simulink model "Progetto_3B_simulink"  (R2019b)
settings: Solver=VariableStepAuto  StartTime=0.0  StopTime=10.0  RelTol=1e-3
values from neighbouring files (symbols this model uses):
  A_n = 0.05    [Progetto_3B.m]
  C_d = (2.2*pi^2)    (= 21.7131296824)    [Progetto_3B.m]
  D = 0    [Progetto_3B.m]
  eta = 0.65    [Progetto_3B.m]
  omega_n = 1500    [Progetto_3B.m]
  R_0 = 35    [Progetto_3B.m]
  u_ = ((x_1/(x_2*abs(x_2))- R_0) / C_d); u_    [Progetto_3B.m]
  x_1 = 10    [Progetto_3B.m]
  x_2 = 5    [Progetto_3B.m]
  y_notlin = -eta*x_1*x_2    (= -32.5)    [Progetto_3B.m]
undefined symbols (not defined in the file or in its folder): N
libraries: cstblocks x2
settings Model: Creator=Hiari  LastModifiedBy=Hiari

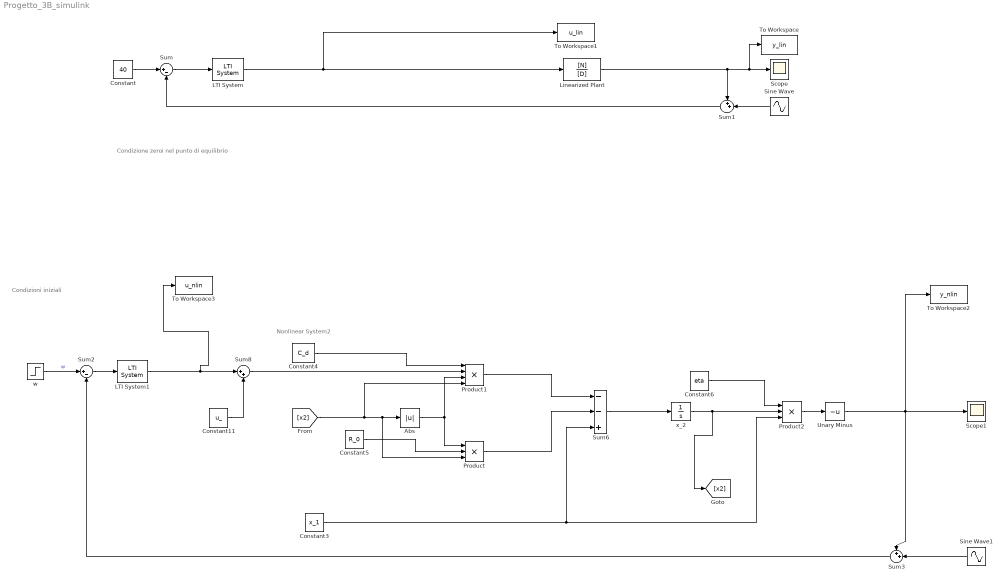
== system Progetto_3B_simulink ==
  note: Nonlinear
      | System2
  note: Condizione zeroi nel punto di equilibrio
  note: Condizioni iniziali
  Abs : Abs
  Constant : Constant  Value=40
  Constant11 : Constant  Value=u_
  Constant3 : Constant  Value=x_1
  Constant4 : Constant  Value=C_d  VectorParams1D=off
  Constant5 : Constant  Value=R_0
  Constant6 : Constant  Value=eta
  LTI System : cstblocks/LTI System  sys=R  IC=[]
  LTI System1 : cstblocks/LTI System  sys=R  IC=[]
  Linearized Plant : TransferFcn  Numerator=[N]  Denominator=[D]
  Product : Product  Inputs=3
  Product1 : Product  Inputs=4
  Product2 : Product  Inputs=3
  Scope : Scope
  Scope1 : Scope
  Sine Wave : Sin  Amplitude=A_n  Frequency=omega_n  SampleTime=0
  Sine Wave1 : Sin  Amplitude=A_n  Frequency=omega_n  SampleTime=0
  Sum : Sum  Inputs=|+-
  Sum1 : Sum  Inputs=++|
  Sum2 : Sum  Inputs=|+-
  Sum3 : Sum  Inputs=++|
  Sum6 : Sum  Inputs=--+
  Sum8 : Sum  Inputs=|++
  To Workspace : ToWorkspace  VariableName=y_lin  SaveFormat=Timeseries  SampleTime=-1
  To Workspace1 : ToWorkspace  VariableName=u_lin  SaveFormat=Timeseries  SampleTime=-1
  To Workspace2 : ToWorkspace  VariableName=y_nlin  SaveFormat=Timeseries  SampleTime=-1
  To Workspace3 : ToWorkspace  VariableName=u_nlin  SaveFormat=Timeseries  SampleTime=-1
  Unary Minus : UnaryMinus
  w : Step  Time=2  Before=y_notlin  After=y_notlin + 0.02  SampleTime=0
  "x_2 " : Integrator  InitialCondition=x_2
  wires:
  Linearized Plant/1 -> To Workspace/1, Scope/1, Sum1/1
  LTI System/1 -> To Workspace1/1, Linearized Plant/1
  Sum/1 -> LTI System/1
  Sine Wave/1 -> Sum1/2
  Sum1/1 -> Sum/2
  Constant/1 -> Sum/1
  Sum2/1 -> LTI System1/1
  Sum3/1 -> Sum2/2
  Constant3/1 -> Product2/3, Sum6/3
  Product2/1 -> Unary Minus/1
  Constant6/1 -> Product2/1
  Constant5/1 -> Product/2
  Abs/1 -> Product/1, Product1/3
  [x2] -> Abs/1, Product/3, Product1/4
  Sum6/1 -> "x_2 "/1
  Product/1 -> Sum6/2
  Product1/1 -> Sum6/1
  Constant4/1 -> Product1/1
  LTI System1/1 -> Sum8/1, To Workspace3/1
  "x_2 "/1 -> [x2], Product2/2
  Sum8/1 -> Product1/2
  Unary Minus/1 -> Sum3/1, To Workspace2/1, Scope1/1
  Constant11/1 -> Sum8/2
  w/1 -> Sum2/1  "w"
  Sine Wave1/1 -> Sum3/2
